simulink model "HANcoder_E407_CAN_COMM_TEST"  (R2018b)
settings: Solver=FixedStepDiscrete  StartTime=0.0  StopTime=1  FixedStep=0.01  RelTol=1e-3
PreLoadFcn:
  | librarySetup
  | eval([bdroot,'_startup']) %Calling [modelName]_startup.m
values from neighbouring files (symbols this model uses):
  HANtuneOverride = Simulink.Parameter    [HANcoder_E407_CAN_COMM_TEST_startup.m]    (also in HANcoder_E407_TTA_Controller_v3_startup.m; HANcoder_E407_TTA_Template_startup.m; HANcoder_Olimexino_startup.m)
  ID_CAN1_const = 24    [HANcoder_E407_CAN_COMM_TEST_startup.m]
  ID_CAN2_const = 24    [HANcoder_E407_CAN_COMM_TEST_startup.m]
  precision_CAN1 = Simulink.Parameter    [HANcoder_E407_CAN_COMM_TEST_startup.m]
  precision_CAN2 = Simulink.Parameter    [HANcoder_E407_CAN_COMM_TEST_startup.m]
  Rx_ID_CAN1 = Simulink.Parameter    [HANcoder_E407_CAN_COMM_TEST_startup.m]
  Rx_ID_CAN2 = Simulink.Parameter    [HANcoder_E407_CAN_COMM_TEST_startup.m]
  Tx_Buffer_1_CAN1 = Simulink.Parameter    [HANcoder_E407_CAN_COMM_TEST_startup.m]
  Tx_Buffer_1_CAN2 = Simulink.Parameter    [HANcoder_E407_CAN_COMM_TEST_startup.m]
  Tx_Buffer_2_CAN1 = Simulink.Parameter    [HANcoder_E407_CAN_COMM_TEST_startup.m]
  Tx_Buffer_2_CAN2 = Simulink.Parameter    [HANcoder_E407_CAN_COMM_TEST_startup.m]
  Tx_Buffer_3_CAN1 = Simulink.Parameter    [HANcoder_E407_CAN_COMM_TEST_startup.m]
  Tx_Buffer_3_CAN2 = Simulink.Parameter    [HANcoder_E407_CAN_COMM_TEST_startup.m]
  Tx_Buffer_4_CAN1 = Simulink.Parameter    [HANcoder_E407_CAN_COMM_TEST_startup.m]
  Tx_Buffer_4_CAN2 = Simulink.Parameter    [HANcoder_E407_CAN_COMM_TEST_startup.m]
  Tx_Buffer_5_CAN1 = Simulink.Parameter    [HANcoder_E407_CAN_COMM_TEST_startup.m]
  Tx_Buffer_5_CAN2 = Simulink.Parameter    [HANcoder_E407_CAN_COMM_TEST_startup.m]
  Tx_Buffer_6_CAN1 = Simulink.Parameter    [HANcoder_E407_CAN_COMM_TEST_startup.m]
  Tx_Buffer_6_CAN2 = Simulink.Parameter    [HANcoder_E407_CAN_COMM_TEST_startup.m]
  Tx_Buffer_7_CAN1 = Simulink.Parameter    [HANcoder_E407_CAN_COMM_TEST_startup.m]
  Tx_Buffer_7_CAN2 = Simulink.Parameter    [HANcoder_E407_CAN_COMM_TEST_startup.m]
  Tx_Buffer_8_CAN1 = Simulink.Parameter    [HANcoder_E407_CAN_COMM_TEST_startup.m]
  Tx_Buffer_8_CAN2 = Simulink.Parameter    [HANcoder_E407_CAN_COMM_TEST_startup.m]
  Tx_ID_CAN1 = Simulink.Parameter    [HANcoder_E407_CAN_COMM_TEST_startup.m]
  Tx_ID_CAN2 = Simulink.Parameter    [HANcoder_E407_CAN_COMM_TEST_startup.m]
  Tx_Max_CAN1 = Simulink.Parameter    [HANcoder_E407_CAN_COMM_TEST_startup.m]
  Tx_Max_CAN2 = Simulink.Parameter    [HANcoder_E407_CAN_COMM_TEST_startup.m]
  Tx_Min_CAN1 = Simulink.Parameter    [HANcoder_E407_CAN_COMM_TEST_startup.m]
  Tx_Min_CAN2 = Simulink.Parameter    [HANcoder_E407_CAN_COMM_TEST_startup.m]
libraries: hdlsllib x48, HANcoder_STM32_Target x13, simulink x2
(part 2 of 3)

== system HANcoder_E407_CAN_COMM_TEST/HANcoder STM32 Target - E407-STM32 algorithm/Rx CAN/uint8_2float4 ==
  precision : Inport
  value : Inport  Port=2
  Bit Shift : hdlsllib/Logic and Bit Operations/Bit Shift  mode=Shift Right Logical  N=7
      settings: SourceProductName=HDL Coder  SourceProductBaseCode=HD
  Bit Shift1 : hdlsllib/Logic and Bit Operations/Bit Shift  mode=Shift Left Logical  N=7
      settings: SourceProductName=HDL Coder  SourceProductBaseCode=HD
  Cast1 : DataTypeConversion  OutDataTypeStr=double
  Constant1 : Constant  Value=2
  Constant2 : Constant  Value=2
  Display{1..5} (5 alike) : Display
  Divide : Product  Inputs=*/
  Fix1 : Rounding  Operator=fix
  Gain : Gain  Gain=-1
  Gain1 : Gain  Gain=-1
  Minus : Sum  Inputs=-+
  Minus1 : Sum  Inputs=+-
  Minus2 : Sum
  Multiply : Product
  Multiply1 : Product
  Power : Math  Priority=5  Operator=pow  SaturateOnIntegerOverflow=on
  Power1 : Math  Priority=5  Operator=pow  SaturateOnIntegerOverflow=on
  Switch : Switch  Criteria=u2 > Threshold
  decoded : Outport
  wires:
  Bit Shift1/1 -> Minus/1
  [prec_pow] -> Multiply1/2
  [prec_pow] -> Divide/2
  Power1/1 -> [prec_pow]
  Constant2/1 -> Power1/1
  precision/1 -> [precision], Power1/2
  Cast1/1 -> Minus/2
  Divide/1 -> Fix1/1
  Switch/1 -> decoded/1, Display3/1
  Gain1/1 -> Switch/1
  Minus2/1 -> Switch/3, Gain1/1
  Multiply/1 -> Minus2/1
  [precision] -> Gain/1
  Power/1 -> Multiply/2
  Gain/1 -> Power/2
  Constant1/1 -> Power/1
  Minus1/1 -> Multiply/1, Display5/1
  Multiply1/1 -> Minus1/2
  Fix1/1 -> Multiply1/1, Display4/1, Minus2/2
  Minus/1 -> Minus1/1, Display2/1, Divide/1
  value/1 -> Bit Shift/1, Cast1/1
  Bit Shift/1 -> Display1/1, Switch/2, Bit Shift1/1

== system HANcoder_E407_CAN_COMM_TEST/HANcoder STM32 Target - E407-STM32 algorithm/Rx CAN/uint8_2float5 ==
  precision : Inport
  value : Inport  Port=2
  Bit Shift : hdlsllib/Logic and Bit Operations/Bit Shift  mode=Shift Right Logical  N=7
      settings: SourceProductName=HDL Coder  SourceProductBaseCode=HD
  Bit Shift1 : hdlsllib/Logic and Bit Operations/Bit Shift  mode=Shift Left Logical  N=7
      settings: SourceProductName=HDL Coder  SourceProductBaseCode=HD
  Cast1 : DataTypeConversion  OutDataTypeStr=double
  Constant1 : Constant  Value=2
  Constant2 : Constant  Value=2
  Display{1..5} (5 alike) : Display
  Divide : Product  Inputs=*/
  Fix1 : Rounding  Operator=fix
  Gain : Gain  Gain=-1
  Gain1 : Gain  Gain=-1
  Minus : Sum  Inputs=-+
  Minus1 : Sum  Inputs=+-
  Minus2 : Sum
  Multiply : Product
  Multiply1 : Product
  Power : Math  Priority=5  Operator=pow  SaturateOnIntegerOverflow=on
  Power1 : Math  Priority=5  Operator=pow  SaturateOnIntegerOverflow=on
  Switch : Switch  Criteria=u2 > Threshold
  decoded : Outport
  wires:
  Bit Shift/1 -> Bit Shift1/1, Switch/2, Display1/1
  value/1 -> Cast1/1, Bit Shift/1
  Minus/1 -> Divide/1, Display2/1, Minus1/1
  Fix1/1 -> Minus2/2, Display4/1, Multiply1/1
  Multiply1/1 -> Minus1/2
  Minus1/1 -> Display5/1, Multiply/1
  Constant1/1 -> Power/1
  Gain/1 -> Power/2
  Power/1 -> Multiply/2
  [precision] -> Gain/1
  Multiply/1 -> Minus2/1
  Minus2/1 -> Gain1/1, Switch/3
  Gain1/1 -> Switch/1
  Switch/1 -> Display3/1, decoded/1
  Divide/1 -> Fix1/1
  Cast1/1 -> Minus/2
  precision/1 -> Power1/2, [precision]
  Constant2/1 -> Power1/1
  Power1/1 -> [prec_pow]
  [prec_pow] -> Divide/2
  [prec_pow] -> Multiply1/2
  Bit Shift1/1 -> Minus/1

== system HANcoder_E407_CAN_COMM_TEST/HANcoder STM32 Target - E407-STM32 algorithm/Rx CAN/uint8_2float6 ==
  precision : Inport
  value : Inport  Port=2
  Bit Shift : hdlsllib/Logic and Bit Operations/Bit Shift  mode=Shift Right Logical  N=7
      settings: SourceProductName=HDL Coder  SourceProductBaseCode=HD
  Bit Shift1 : hdlsllib/Logic and Bit Operations/Bit Shift  mode=Shift Left Logical  N=7
      settings: SourceProductName=HDL Coder  SourceProductBaseCode=HD
  Cast1 : DataTypeConversion  OutDataTypeStr=double
  Constant1 : Constant  Value=2
  Constant2 : Constant  Value=2
  Display{1..5} (5 alike) : Display
  Divide : Product  Inputs=*/
  Fix1 : Rounding  Operator=fix
  Gain : Gain  Gain=-1
  Gain1 : Gain  Gain=-1
  Minus : Sum  Inputs=-+
  Minus1 : Sum  Inputs=+-
  Minus2 : Sum
  Multiply : Product
  Multiply1 : Product
  Power : Math  Priority=5  Operator=pow  SaturateOnIntegerOverflow=on
  Power1 : Math  Priority=5  Operator=pow  SaturateOnIntegerOverflow=on
  Switch : Switch  Criteria=u2 > Threshold
  decoded : Outport
  wires:
  Bit Shift1/1 -> Minus/1
  [prec_pow] -> Multiply1/2
  [prec_pow] -> Divide/2
  Power1/1 -> [prec_pow]
  Constant2/1 -> Power1/1
  precision/1 -> [precision], Power1/2
  Cast1/1 -> Minus/2
  Divide/1 -> Fix1/1
  Switch/1 -> decoded/1, Display3/1
  Gain1/1 -> Switch/1
  Minus2/1 -> Switch/3, Gain1/1
  Multiply/1 -> Minus2/1
  [precision] -> Gain/1
  Power/1 -> Multiply/2
  Gain/1 -> Power/2
  Constant1/1 -> Power/1
  Minus1/1 -> Multiply/1, Display5/1
  Multiply1/1 -> Minus1/2
  Fix1/1 -> Multiply1/1, Display4/1, Minus2/2
  Minus/1 -> Minus1/1, Display2/1, Divide/1
  value/1 -> Bit Shift/1, Cast1/1
  Bit Shift/1 -> Display1/1, Switch/2, Bit Shift1/1

== system HANcoder_E407_CAN_COMM_TEST/HANcoder STM32 Target - E407-STM32 algorithm/Rx CAN/uint8_2float7 ==
  precision : Inport
  value : Inport  Port=2
  Bit Shift : hdlsllib/Logic and Bit Operations/Bit Shift  mode=Shift Right Logical  N=7
      settings: SourceProductName=HDL Coder  SourceProductBaseCode=HD
  Bit Shift1 : hdlsllib/Logic and Bit Operations/Bit Shift  mode=Shift Left Logical  N=7
      settings: SourceProductName=HDL Coder  SourceProductBaseCode=HD
  Cast1 : DataTypeConversion  OutDataTypeStr=double
  Constant1 : Constant  Value=2
  Constant2 : Constant  Value=2
  Display{1..5} (5 alike) : Display
  Divide : Product  Inputs=*/
  Fix1 : Rounding  Operator=fix
  Gain : Gain  Gain=-1
  Gain1 : Gain  Gain=-1
  Minus : Sum  Inputs=-+
  Minus1 : Sum  Inputs=+-
  Minus2 : Sum
  Multiply : Product
  Multiply1 : Product
  Power : Math  Priority=5  Operator=pow  SaturateOnIntegerOverflow=on
  Power1 : Math  Priority=5  Operator=pow  SaturateOnIntegerOverflow=on
  Switch : Switch  Criteria=u2 > Threshold
  decoded : Outport
  wires:
  Bit Shift/1 -> Bit Shift1/1, Switch/2, Display1/1
  value/1 -> Cast1/1, Bit Shift/1
  Minus/1 -> Divide/1, Display2/1, Minus1/1
  Fix1/1 -> Minus2/2, Display4/1, Multiply1/1
  Multiply1/1 -> Minus1/2
  Minus1/1 -> Display5/1, Multiply/1
  Constant1/1 -> Power/1
  Gain/1 -> Power/2
  Power/1 -> Multiply/2
  [precision] -> Gain/1
  Multiply/1 -> Minus2/1
  Minus2/1 -> Gain1/1, Switch/3
  Gain1/1 -> Switch/1
  Switch/1 -> Display3/1, decoded/1
  Divide/1 -> Fix1/1
  Cast1/1 -> Minus/2
  precision/1 -> Power1/2, [precision]
  Constant2/1 -> Power1/1
  Power1/1 -> [prec_pow]
  [prec_pow] -> Divide/2
  [prec_pow] -> Multiply1/2
  Bit Shift1/1 -> Minus/1

== system HANcoder_E407_CAN_COMM_TEST/HANcoder STM32 Target - E407-STM32 algorithm/Rx CAN/uint8_2float8 ==
  precision : Inport
  value : Inport  Port=2
  Bit Shift : hdlsllib/Logic and Bit Operations/Bit Shift  mode=Shift Right Logical  N=7
      settings: SourceProductName=HDL Coder  SourceProductBaseCode=HD
  Bit Shift1 : hdlsllib/Logic and Bit Operations/Bit Shift  mode=Shift Left Logical  N=7
      settings: SourceProductName=HDL Coder  SourceProductBaseCode=HD
  Cast1 : DataTypeConversion  OutDataTypeStr=double
  Constant1 : Constant  Value=2
  Constant2 : Constant  Value=2
  Display{1..5} (5 alike) : Display
  Divide : Product  Inputs=*/
  Fix1 : Rounding  Operator=fix
  Gain : Gain  Gain=-1
  Gain1 : Gain  Gain=-1
  Minus : Sum  Inputs=-+
  Minus1 : Sum  Inputs=+-
  Minus2 : Sum
  Multiply : Product
  Multiply1 : Product
  Power : Math  Priority=5  Operator=pow  SaturateOnIntegerOverflow=on
  Power1 : Math  Priority=5  Operator=pow  SaturateOnIntegerOverflow=on
  Switch : Switch  Criteria=u2 > Threshold
  decoded : Outport
  wires:
  Bit Shift/1 -> Bit Shift1/1, Switch/2, Display1/1
  value/1 -> Cast1/1, Bit Shift/1
  Minus/1 -> Divide/1, Display2/1, Minus1/1
  Fix1/1 -> Minus2/2, Display4/1, Multiply1/1
  Multiply1/1 -> Minus1/2
  Minus1/1 -> Display5/1, Multiply/1
  Constant1/1 -> Power/1
  Gain/1 -> Power/2
  Power/1 -> Multiply/2
  [precision] -> Gain/1
  Multiply/1 -> Minus2/1
  Minus2/1 -> Gain1/1, Switch/3
  Gain1/1 -> Switch/1
  Switch/1 -> Display3/1, decoded/1
  Divide/1 -> Fix1/1
  Cast1/1 -> Minus/2
  precision/1 -> Power1/2, [precision]
  Constant2/1 -> Power1/1
  Power1/1 -> [prec_pow]
  [prec_pow] -> Divide/2
  [prec_pow] -> Multiply1/2
  Bit Shift1/1 -> Minus/1

== system HANcoder_E407_CAN_COMM_TEST/HANcoder STM32 Target - E407-STM32 algorithm/Rx CAN/uint8_2float9 ==
  precision : Inport
  value : Inport  Port=2
  Bit Shift : hdlsllib/Logic and Bit Operations/Bit Shift  mode=Shift Right Logical  N=7
      settings: SourceProductName=HDL Coder  SourceProductBaseCode=HD
  Bit Shift1 : hdlsllib/Logic and Bit Operations/Bit Shift  mode=Shift Left Logical  N=7
      settings: SourceProductName=HDL Coder  SourceProductBaseCode=HD
  Cast1 : DataTypeConversion  OutDataTypeStr=double
  Constant1 : Constant  Value=2
  Constant2 : Constant  Value=2
  Display{1..5} (5 alike) : Display
  Divide : Product  Inputs=*/
  Fix1 : Rounding  Operator=fix
  Gain : Gain  Gain=-1
  Gain1 : Gain  Gain=-1
  Minus : Sum  Inputs=-+
  Minus1 : Sum  Inputs=+-
  Minus2 : Sum
  Multiply : Product
  Multiply1 : Product
  Power : Math  Priority=5  Operator=pow  SaturateOnIntegerOverflow=on
  Power1 : Math  Priority=5  Operator=pow  SaturateOnIntegerOverflow=on
  Switch : Switch  Criteria=u2 > Threshold
  decoded : Outport
  wires:
  Bit Shift/1 -> Bit Shift1/1, Switch/2, Display1/1
  value/1 -> Cast1/1, Bit Shift/1
  Minus/1 -> Divide/1, Display2/1, Minus1/1
  Fix1/1 -> Minus2/2, Display4/1, Multiply1/1
  Multiply1/1 -> Minus1/2
  Minus1/1 -> Display5/1, Multiply/1
  Constant1/1 -> Power/1
  Gain/1 -> Power/2
  Power/1 -> Multiply/2
  [precision] -> Gain/1
  Multiply/1 -> Minus2/1
  Minus2/1 -> Gain1/1, Switch/3
  Gain1/1 -> Switch/1
  Switch/1 -> Display3/1, decoded/1
  Divide/1 -> Fix1/1
  Cast1/1 -> Minus/2
  precision/1 -> Power1/2, [precision]
  Constant2/1 -> Power1/1
  Power1/1 -> [prec_pow]
  [prec_pow] -> Divide/2
  [prec_pow] -> Multiply1/2
  Bit Shift1/1 -> Minus/1

== system HANcoder_E407_CAN_COMM_TEST/HANcoder STM32 Target - E407-STM32 algorithm/Tx CAN/CAN send ==
  In1 : Inport
  In2 : Inport  Port=2
  In3 : Inport  Port=3
  In4 : Inport  Port=4
  In5 : Inport  Port=5
  In6 : Inport  Port=6
  In7 : Inport  Port=7
  In8 : Inport  Port=8
  In9 : Inport  Port=9
  S-Function : M-S-Function  FunctionName=sfcn_can_send  Parameters=tsamp, canBus, frameType, inputNumber, dataType, byteOrder
  wires:
  In1/1 -> S-Function/1
  In2/1 -> S-Function/2
  In3/1 -> S-Function/3
  In4/1 -> S-Function/4
  In5/1 -> S-Function/5
  In6/1 -> S-Function/6
  In7/1 -> S-Function/7
  In8/1 -> S-Function/8
  In9/1 -> S-Function/9

== system HANcoder_E407_CAN_COMM_TEST/HANcoder STM32 Target - E407-STM32 algorithm/Tx CAN/CAN send1 ==
  In1 : Inport
  In2 : Inport  Port=2
  In3 : Inport  Port=3
  In4 : Inport  Port=4
  In5 : Inport  Port=5
  In6 : Inport  Port=6
  In7 : Inport  Port=7
  In8 : Inport  Port=8
  In9 : Inport  Port=9
  S-Function : M-S-Function  FunctionName=sfcn_can_send  Parameters=tsamp, canBus, frameType, inputNumber, dataType, byteOrder
  wires:
  In9/1 -> S-Function/9
  In8/1 -> S-Function/8
  In7/1 -> S-Function/7
  In6/1 -> S-Function/6
  In5/1 -> S-Function/5
  In4/1 -> S-Function/4
  In3/1 -> S-Function/3
  In2/1 -> S-Function/2
  In1/1 -> S-Function/1

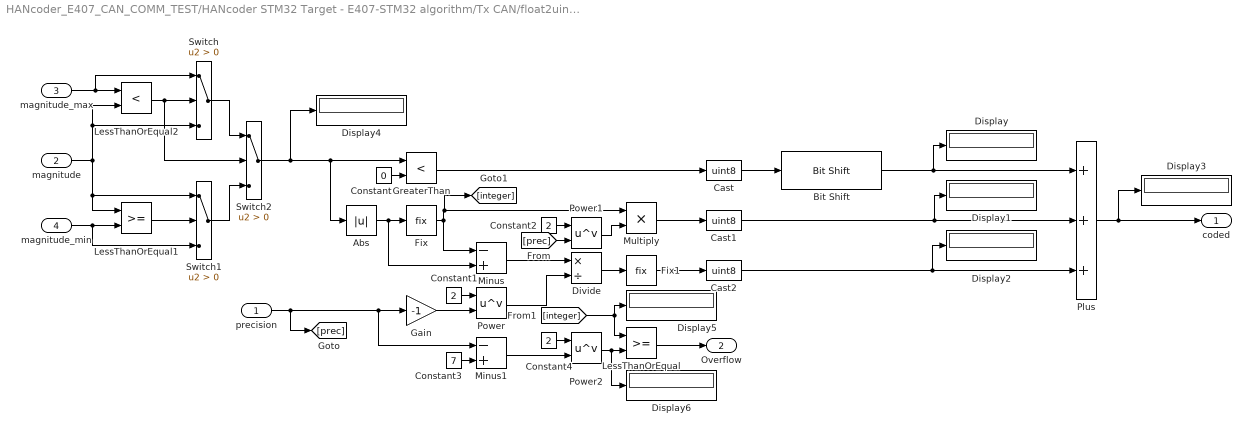
== system HANcoder_E407_CAN_COMM_TEST/HANcoder STM32 Target - E407-STM32 algorithm/Tx CAN/float2uint1 ==
  precision : Inport
  magnitude : Inport  Port=2
  magnitude_max : Inport  Port=3
  magnitude_min : Inport  Port=4
  Abs : Abs
  Bit Shift : hdlsllib/Logic and Bit Operations/Bit Shift  mode=Shift Left Logical  N=7
      settings: SourceProductName=HDL Coder  SourceProductBaseCode=HD
  Cast : DataTypeConversion  OutDataTypeStr=uint8
  Cast1 : DataTypeConversion  OutDataTypeStr=uint8
  Cast2 : DataTypeConversion  OutDataTypeStr=uint8
  Constant : Constant  Value=0
  Constant1 : Constant  Value=2
  Constant2 : Constant  Value=2
  Constant3 : Constant  Value=7
  Constant4 : Constant  Value=2
  Display{,1..6} (7 alike) : Display
  Divide : Product  Inputs=*/
  Fix : Rounding  Priority=3  Operator=fix
  Fix1 : Rounding  Priority=6  Operator=fix
  Gain : Gain  Gain=-1
  GreaterThan : RelationalOperator  Priority=2  Operator=<  OutDataTypeStr=boolean  RndMeth=Simplest
  LessThanOrEqual : RelationalOperator  OutDataTypeStr=boolean  RndMeth=Simplest
  LessThanOrEqual1 : RelationalOperator  OutDataTypeStr=boolean  RndMeth=Simplest
  LessThanOrEqual2 : RelationalOperator  Operator=<  OutDataTypeStr=boolean  RndMeth=Simplest
  Minus : Sum  Priority=4  Inputs=-+
  Minus1 : Sum  Priority=4  Inputs=-+
  Multiply : Product
  Plus : Sum  Priority=10  Inputs=+++
  Power : Math  Priority=5  Operator=pow  SaturateOnIntegerOverflow=on
  Power1 : Math  Priority=5  Operator=pow  SaturateOnIntegerOverflow=on
  Power2 : Math  Priority=5  Operator=pow  SaturateOnIntegerOverflow=on
  Switch : Switch  Criteria=u2 > Threshold
  Switch1 : Switch  Criteria=u2 > Threshold
  Switch2 : Switch  Criteria=u2 > Threshold
  coded : Outport
  Overflow : Outport  Port=2
  wires:
  Constant/1 -> GreaterThan/2
  Switch2/1 -> Display4/1, Abs/1, GreaterThan/1
  Abs/1 -> Minus/2, Fix/1
  GreaterThan/1 -> Cast/1
  Fix/1 -> [integer], Multiply/1, Minus/1
  Minus/1 -> Divide/1
  Cast/1 -> Bit Shift/1
  Bit Shift/1 -> Display/1, Plus/1
  Cast1/1 -> Display1/1, Plus/2
  Constant1/1 -> Power/1
  Gain/1 -> Power/2
  Power/1 -> Divide/2
  Divide/1 -> Fix1/1
  Fix1/1 -> Cast2/1
  Cast2/1 -> Display2/1, Plus/3
  Constant2/1 -> Power1/1
  Power1/1 -> Multiply/2
  precision/1 -> [prec], Minus1/1, Gain/1
  Multiply/1 -> Cast1/1
  [prec] -> Power1/2
  Constant3/1 -> Minus1/2
  Minus1/1 -> Power2/2
  Constant4/1 -> Power2/1
  Power2/1 -> Display6/1, LessThanOrEqual/2
  LessThanOrEqual/1 -> Overflow/1
  Plus/1 -> coded/1, Display3/1
  magnitude/1 -> LessThanOrEqual1/1, Switch1/1, LessThanOrEqual2/2, Switch/3
  magnitude_min/1 -> LessThanOrEqual1/2, Switch1/3
  magnitude_max/1 -> Switch/1, LessThanOrEqual2/1
  LessThanOrEqual2/1 -> Switch2/2, Switch/2
  LessThanOrEqual1/1 -> Switch1/2
  Switch/1 -> Switch2/1
  Switch1/1 -> Switch2/3
  [integer] -> Display5/1, LessThanOrEqual/1

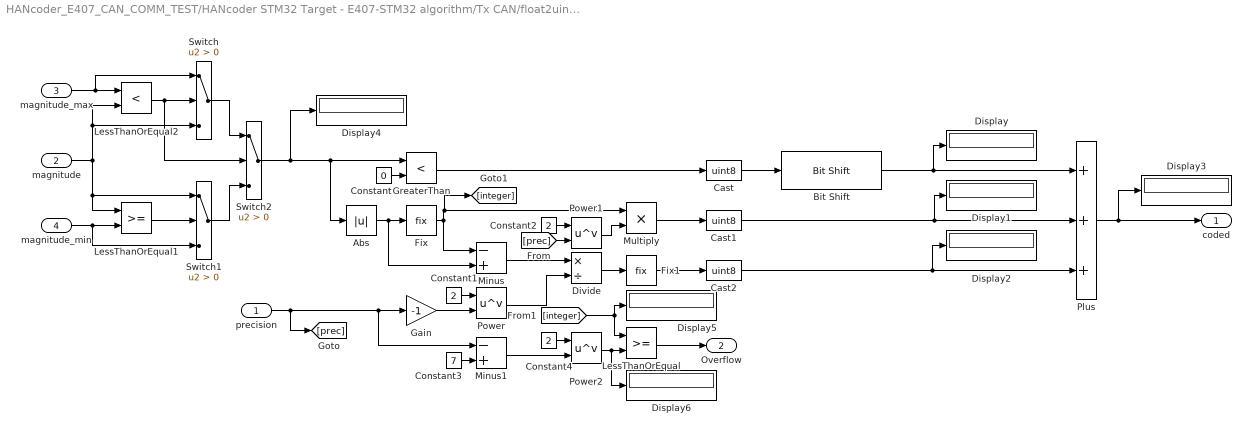
== system HANcoder_E407_CAN_COMM_TEST/HANcoder STM32 Target - E407-STM32 algorithm/Tx CAN/float2uint10 ==
  precision : Inport
  magnitude : Inport  Port=2
  magnitude_max : Inport  Port=3
  magnitude_min : Inport  Port=4
  Abs : Abs
  Bit Shift : hdlsllib/Logic and Bit Operations/Bit Shift  mode=Shift Left Logical  N=7
      settings: SourceProductName=HDL Coder  SourceProductBaseCode=HD
  Cast : DataTypeConversion  OutDataTypeStr=uint8
  Cast1 : DataTypeConversion  OutDataTypeStr=uint8
  Cast2 : DataTypeConversion  OutDataTypeStr=uint8
  Constant : Constant  Value=0
  Constant1 : Constant  Value=2
  Constant2 : Constant  Value=2
  Constant3 : Constant  Value=7
  Constant4 : Constant  Value=2
  Display{,1..6} (7 alike) : Display
  Divide : Product  Inputs=*/
  Fix : Rounding  Priority=3  Operator=fix
  Fix1 : Rounding  Priority=6  Operator=fix
  Gain : Gain  Gain=-1
  GreaterThan : RelationalOperator  Priority=2  Operator=<  OutDataTypeStr=boolean  RndMeth=Simplest
  LessThanOrEqual : RelationalOperator  OutDataTypeStr=boolean  RndMeth=Simplest
  LessThanOrEqual1 : RelationalOperator  OutDataTypeStr=boolean  RndMeth=Simplest
  LessThanOrEqual2 : RelationalOperator  Operator=<  OutDataTypeStr=boolean  RndMeth=Simplest
  Minus : Sum  Priority=4  Inputs=-+
  Minus1 : Sum  Priority=4  Inputs=-+
  Multiply : Product
  Plus : Sum  Priority=10  Inputs=+++
  Power : Math  Priority=5  Operator=pow  SaturateOnIntegerOverflow=on
  Power1 : Math  Priority=5  Operator=pow  SaturateOnIntegerOverflow=on
  Power2 : Math  Priority=5  Operator=pow  SaturateOnIntegerOverflow=on
  Switch : Switch  Criteria=u2 > Threshold
  Switch1 : Switch  Criteria=u2 > Threshold
  Switch2 : Switch  Criteria=u2 > Threshold
  coded : Outport
  Overflow : Outport  Port=2
  wires:
  Constant/1 -> GreaterThan/2
  Switch2/1 -> Display4/1, Abs/1, GreaterThan/1
  Abs/1 -> Minus/2, Fix/1
  GreaterThan/1 -> Cast/1
  Fix/1 -> [integer], Multiply/1, Minus/1
  Minus/1 -> Divide/1
  Cast/1 -> Bit Shift/1
  Bit Shift/1 -> Display/1, Plus/1
  Cast1/1 -> Display1/1, Plus/2
  Constant1/1 -> Power/1
  Gain/1 -> Power/2
  Power/1 -> Divide/2
  Divide/1 -> Fix1/1
  Fix1/1 -> Cast2/1
  Cast2/1 -> Display2/1, Plus/3
  Constant2/1 -> Power1/1
  Power1/1 -> Multiply/2
  precision/1 -> [prec], Minus1/1, Gain/1
  Multiply/1 -> Cast1/1
  [prec] -> Power1/2
  Constant3/1 -> Minus1/2
  Minus1/1 -> Power2/2
  Constant4/1 -> Power2/1
  Power2/1 -> Display6/1, LessThanOrEqual/2
  LessThanOrEqual/1 -> Overflow/1
  Plus/1 -> coded/1, Display3/1
  magnitude/1 -> LessThanOrEqual1/1, Switch1/1, LessThanOrEqual2/2, Switch/3
  magnitude_min/1 -> LessThanOrEqual1/2, Switch1/3
  magnitude_max/1 -> Switch/1, LessThanOrEqual2/1
  LessThanOrEqual2/1 -> Switch2/2, Switch/2
  LessThanOrEqual1/1 -> Switch1/2
  Switch/1 -> Switch2/1
  Switch1/1 -> Switch2/3
  [integer] -> Display5/1, LessThanOrEqual/1

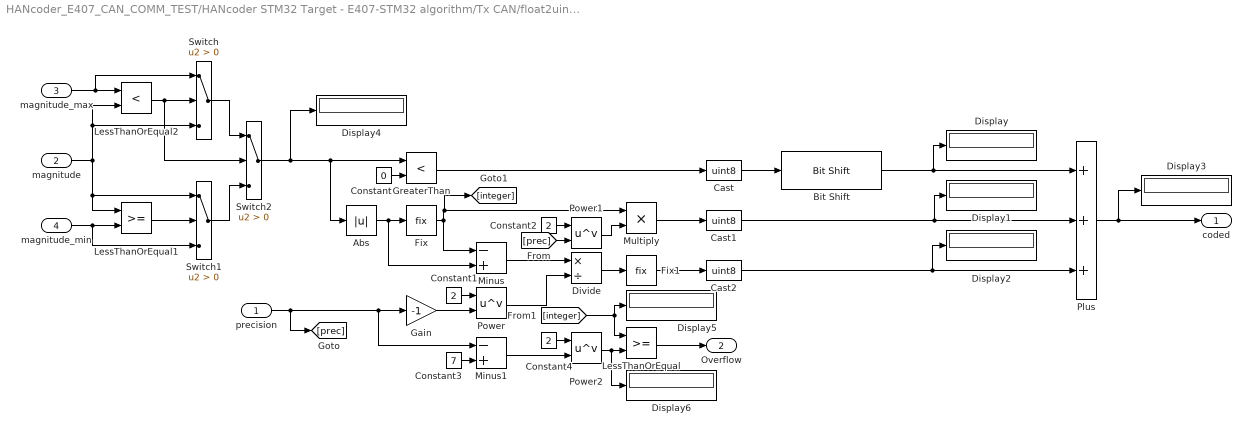
== system HANcoder_E407_CAN_COMM_TEST/HANcoder STM32 Target - E407-STM32 algorithm/Tx CAN/float2uint11 ==
  precision : Inport
  magnitude : Inport  Port=2
  magnitude_max : Inport  Port=3
  magnitude_min : Inport  Port=4
  Abs : Abs
  Bit Shift : hdlsllib/Logic and Bit Operations/Bit Shift  mode=Shift Left Logical  N=7
      settings: SourceProductName=HDL Coder  SourceProductBaseCode=HD
  Cast : DataTypeConversion  OutDataTypeStr=uint8
  Cast1 : DataTypeConversion  OutDataTypeStr=uint8
  Cast2 : DataTypeConversion  OutDataTypeStr=uint8
  Constant : Constant  Value=0
  Constant1 : Constant  Value=2
  Constant2 : Constant  Value=2
  Constant3 : Constant  Value=7
  Constant4 : Constant  Value=2
  Display{,1..6} (7 alike) : Display
  Divide : Product  Inputs=*/
  Fix : Rounding  Priority=3  Operator=fix
  Fix1 : Rounding  Priority=6  Operator=fix
  Gain : Gain  Gain=-1
  GreaterThan : RelationalOperator  Priority=2  Operator=<  OutDataTypeStr=boolean  RndMeth=Simplest
  LessThanOrEqual : RelationalOperator  OutDataTypeStr=boolean  RndMeth=Simplest
  LessThanOrEqual1 : RelationalOperator  OutDataTypeStr=boolean  RndMeth=Simplest
  LessThanOrEqual2 : RelationalOperator  Operator=<  OutDataTypeStr=boolean  RndMeth=Simplest
  Minus : Sum  Priority=4  Inputs=-+
  Minus1 : Sum  Priority=4  Inputs=-+
  Multiply : Product
  Plus : Sum  Priority=10  Inputs=+++
  Power : Math  Priority=5  Operator=pow  SaturateOnIntegerOverflow=on
  Power1 : Math  Priority=5  Operator=pow  SaturateOnIntegerOverflow=on
  Power2 : Math  Priority=5  Operator=pow  SaturateOnIntegerOverflow=on
  Switch : Switch  Criteria=u2 > Threshold
  Switch1 : Switch  Criteria=u2 > Threshold
  Switch2 : Switch  Criteria=u2 > Threshold
  coded : Outport
  Overflow : Outport  Port=2
  wires:
  [integer] -> LessThanOrEqual/1, Display5/1
  Switch1/1 -> Switch2/3
  Switch/1 -> Switch2/1
  LessThanOrEqual1/1 -> Switch1/2
  LessThanOrEqual2/1 -> Switch/2, Switch2/2
  magnitude_max/1 -> LessThanOrEqual2/1, Switch/1
  magnitude_min/1 -> Switch1/3, LessThanOrEqual1/2
  magnitude/1 -> Switch/3, LessThanOrEqual2/2, Switch1/1, LessThanOrEqual1/1
  Plus/1 -> Display3/1, coded/1
  LessThanOrEqual/1 -> Overflow/1
  Power2/1 -> LessThanOrEqual/2, Display6/1
  Constant4/1 -> Power2/1
  Minus1/1 -> Power2/2
  Constant3/1 -> Minus1/2
  [prec] -> Power1/2
  Multiply/1 -> Cast1/1
  precision/1 -> Gain/1, Minus1/1, [prec]
  Power1/1 -> Multiply/2
  Constant2/1 -> Power1/1
  Cast2/1 -> Plus/3, Display2/1
  Fix1/1 -> Cast2/1
  Divide/1 -> Fix1/1
  Power/1 -> Divide/2
  Gain/1 -> Power/2
  Constant1/1 -> Power/1
  Cast1/1 -> Plus/2, Display1/1
  Bit Shift/1 -> Plus/1, Display/1
  Cast/1 -> Bit Shift/1
  Minus/1 -> Divide/1
  Fix/1 -> Minus/1, Multiply/1, [integer]
  GreaterThan/1 -> Cast/1
  Abs/1 -> Fix/1, Minus/2
  Switch2/1 -> GreaterThan/1, Abs/1, Display4/1
  Constant/1 -> GreaterThan/2

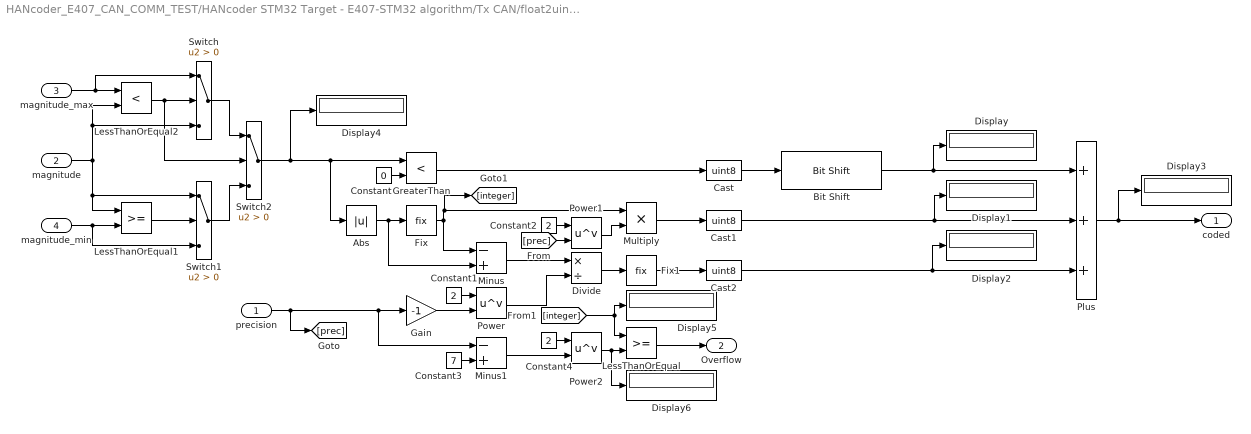
== system HANcoder_E407_CAN_COMM_TEST/HANcoder STM32 Target - E407-STM32 algorithm/Tx CAN/float2uint12 ==
  precision : Inport
  magnitude : Inport  Port=2
  magnitude_max : Inport  Port=3
  magnitude_min : Inport  Port=4
  Abs : Abs
  Bit Shift : hdlsllib/Logic and Bit Operations/Bit Shift  mode=Shift Left Logical  N=7
      settings: SourceProductName=HDL Coder  SourceProductBaseCode=HD
  Cast : DataTypeConversion  OutDataTypeStr=uint8
  Cast1 : DataTypeConversion  OutDataTypeStr=uint8
  Cast2 : DataTypeConversion  OutDataTypeStr=uint8
  Constant : Constant  Value=0
  Constant1 : Constant  Value=2
  Constant2 : Constant  Value=2
  Constant3 : Constant  Value=7
  Constant4 : Constant  Value=2
  Display{,1..6} (7 alike) : Display
  Divide : Product  Inputs=*/
  Fix : Rounding  Priority=3  Operator=fix
  Fix1 : Rounding  Priority=6  Operator=fix
  Gain : Gain  Gain=-1
  GreaterThan : RelationalOperator  Priority=2  Operator=<  OutDataTypeStr=boolean  RndMeth=Simplest
  LessThanOrEqual : RelationalOperator  OutDataTypeStr=boolean  RndMeth=Simplest
  LessThanOrEqual1 : RelationalOperator  OutDataTypeStr=boolean  RndMeth=Simplest
  LessThanOrEqual2 : RelationalOperator  Operator=<  OutDataTypeStr=boolean  RndMeth=Simplest
  Minus : Sum  Priority=4  Inputs=-+
  Minus1 : Sum  Priority=4  Inputs=-+
  Multiply : Product
  Plus : Sum  Priority=10  Inputs=+++
  Power : Math  Priority=5  Operator=pow  SaturateOnIntegerOverflow=on
  Power1 : Math  Priority=5  Operator=pow  SaturateOnIntegerOverflow=on
  Power2 : Math  Priority=5  Operator=pow  SaturateOnIntegerOverflow=on
  Switch : Switch  Criteria=u2 > Threshold
  Switch1 : Switch  Criteria=u2 > Threshold
  Switch2 : Switch  Criteria=u2 > Threshold
  coded : Outport
  Overflow : Outport  Port=2
  wires:
  Constant/1 -> GreaterThan/2
  Switch2/1 -> Display4/1, Abs/1, GreaterThan/1
  Abs/1 -> Minus/2, Fix/1
  GreaterThan/1 -> Cast/1
  Fix/1 -> [integer], Multiply/1, Minus/1
  Minus/1 -> Divide/1
  Cast/1 -> Bit Shift/1
  Bit Shift/1 -> Display/1, Plus/1
  Cast1/1 -> Display1/1, Plus/2
  Constant1/1 -> Power/1
  Gain/1 -> Power/2
  Power/1 -> Divide/2
  Divide/1 -> Fix1/1
  Fix1/1 -> Cast2/1
  Cast2/1 -> Display2/1, Plus/3
  Constant2/1 -> Power1/1
  Power1/1 -> Multiply/2
  precision/1 -> [prec], Minus1/1, Gain/1
  Multiply/1 -> Cast1/1
  [prec] -> Power1/2
  Constant3/1 -> Minus1/2
  Minus1/1 -> Power2/2
  Constant4/1 -> Power2/1
  Power2/1 -> Display6/1, LessThanOrEqual/2
  LessThanOrEqual/1 -> Overflow/1
  Plus/1 -> coded/1, Display3/1
  magnitude/1 -> LessThanOrEqual1/1, Switch1/1, LessThanOrEqual2/2, Switch/3
  magnitude_min/1 -> LessThanOrEqual1/2, Switch1/3
  magnitude_max/1 -> Switch/1, LessThanOrEqual2/1
  LessThanOrEqual2/1 -> Switch2/2, Switch/2
  LessThanOrEqual1/1 -> Switch1/2
  Switch/1 -> Switch2/1
  Switch1/1 -> Switch2/3
  [integer] -> Display5/1, LessThanOrEqual/1

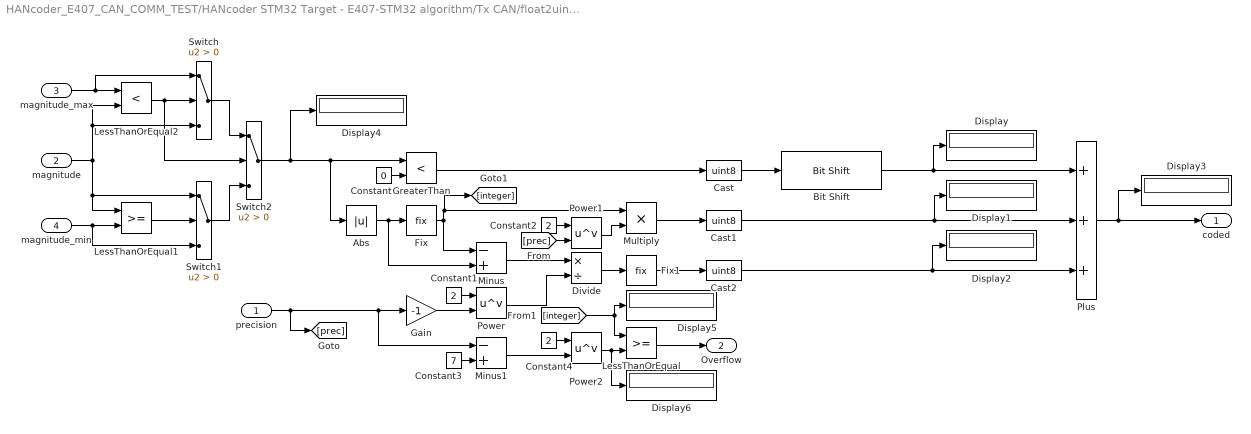
== system HANcoder_E407_CAN_COMM_TEST/HANcoder STM32 Target - E407-STM32 algorithm/Tx CAN/float2uint13 ==
  precision : Inport
  magnitude : Inport  Port=2
  magnitude_max : Inport  Port=3
  magnitude_min : Inport  Port=4
  Abs : Abs
  Bit Shift : hdlsllib/Logic and Bit Operations/Bit Shift  mode=Shift Left Logical  N=7
      settings: SourceProductName=HDL Coder  SourceProductBaseCode=HD
  Cast : DataTypeConversion  OutDataTypeStr=uint8
  Cast1 : DataTypeConversion  OutDataTypeStr=uint8
  Cast2 : DataTypeConversion  OutDataTypeStr=uint8
  Constant : Constant  Value=0
  Constant1 : Constant  Value=2
  Constant2 : Constant  Value=2
  Constant3 : Constant  Value=7
  Constant4 : Constant  Value=2
  Display{,1..6} (7 alike) : Display
  Divide : Product  Inputs=*/
  Fix : Rounding  Priority=3  Operator=fix
  Fix1 : Rounding  Priority=6  Operator=fix
  Gain : Gain  Gain=-1
  GreaterThan : RelationalOperator  Priority=2  Operator=<  OutDataTypeStr=boolean  RndMeth=Simplest
  LessThanOrEqual : RelationalOperator  OutDataTypeStr=boolean  RndMeth=Simplest
  LessThanOrEqual1 : RelationalOperator  OutDataTypeStr=boolean  RndMeth=Simplest
  LessThanOrEqual2 : RelationalOperator  Operator=<  OutDataTypeStr=boolean  RndMeth=Simplest
  Minus : Sum  Priority=4  Inputs=-+
  Minus1 : Sum  Priority=4  Inputs=-+
  Multiply : Product
  Plus : Sum  Priority=10  Inputs=+++
  Power : Math  Priority=5  Operator=pow  SaturateOnIntegerOverflow=on
  Power1 : Math  Priority=5  Operator=pow  SaturateOnIntegerOverflow=on
  Power2 : Math  Priority=5  Operator=pow  SaturateOnIntegerOverflow=on
  Switch : Switch  Criteria=u2 > Threshold
  Switch1 : Switch  Criteria=u2 > Threshold
  Switch2 : Switch  Criteria=u2 > Threshold
  coded : Outport
  Overflow : Outport  Port=2
  wires:
  [integer] -> LessThanOrEqual/1, Display5/1
  Switch1/1 -> Switch2/3
  Switch/1 -> Switch2/1
  LessThanOrEqual1/1 -> Switch1/2
  LessThanOrEqual2/1 -> Switch/2, Switch2/2
  magnitude_max/1 -> LessThanOrEqual2/1, Switch/1
  magnitude_min/1 -> Switch1/3, LessThanOrEqual1/2
  magnitude/1 -> Switch/3, LessThanOrEqual2/2, Switch1/1, LessThanOrEqual1/1
  Plus/1 -> Display3/1, coded/1
  LessThanOrEqual/1 -> Overflow/1
  Power2/1 -> LessThanOrEqual/2, Display6/1
  Constant4/1 -> Power2/1
  Minus1/1 -> Power2/2
  Constant3/1 -> Minus1/2
  [prec] -> Power1/2
  Multiply/1 -> Cast1/1
  precision/1 -> Gain/1, Minus1/1, [prec]
  Power1/1 -> Multiply/2
  Constant2/1 -> Power1/1
  Cast2/1 -> Plus/3, Display2/1
  Fix1/1 -> Cast2/1
  Divide/1 -> Fix1/1
  Power/1 -> Divide/2
  Gain/1 -> Power/2
  Constant1/1 -> Power/1
  Cast1/1 -> Plus/2, Display1/1
  Bit Shift/1 -> Plus/1, Display/1
  Cast/1 -> Bit Shift/1
  Minus/1 -> Divide/1
  Fix/1 -> Minus/1, Multiply/1, [integer]
  GreaterThan/1 -> Cast/1
  Abs/1 -> Fix/1, Minus/2
  Switch2/1 -> GreaterThan/1, Abs/1, Display4/1
  Constant/1 -> GreaterThan/2

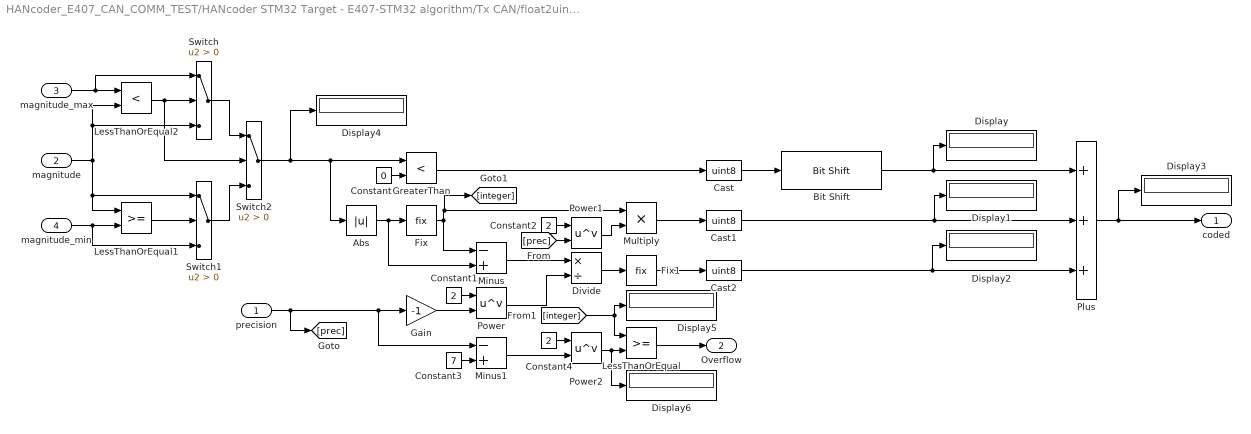
== system HANcoder_E407_CAN_COMM_TEST/HANcoder STM32 Target - E407-STM32 algorithm/Tx CAN/float2uint14 ==
  precision : Inport
  magnitude : Inport  Port=2
  magnitude_max : Inport  Port=3
  magnitude_min : Inport  Port=4
  Abs : Abs
  Bit Shift : hdlsllib/Logic and Bit Operations/Bit Shift  mode=Shift Left Logical  N=7
      settings: SourceProductName=HDL Coder  SourceProductBaseCode=HD
  Cast : DataTypeConversion  OutDataTypeStr=uint8
  Cast1 : DataTypeConversion  OutDataTypeStr=uint8
  Cast2 : DataTypeConversion  OutDataTypeStr=uint8
  Constant : Constant  Value=0
  Constant1 : Constant  Value=2
  Constant2 : Constant  Value=2
  Constant3 : Constant  Value=7
  Constant4 : Constant  Value=2
  Display{,1..6} (7 alike) : Display
  Divide : Product  Inputs=*/
  Fix : Rounding  Priority=3  Operator=fix
  Fix1 : Rounding  Priority=6  Operator=fix
  Gain : Gain  Gain=-1
  GreaterThan : RelationalOperator  Priority=2  Operator=<  OutDataTypeStr=boolean  RndMeth=Simplest
  LessThanOrEqual : RelationalOperator  OutDataTypeStr=boolean  RndMeth=Simplest
  LessThanOrEqual1 : RelationalOperator  OutDataTypeStr=boolean  RndMeth=Simplest
  LessThanOrEqual2 : RelationalOperator  Operator=<  OutDataTypeStr=boolean  RndMeth=Simplest
  Minus : Sum  Priority=4  Inputs=-+
  Minus1 : Sum  Priority=4  Inputs=-+
  Multiply : Product
  Plus : Sum  Priority=10  Inputs=+++
  Power : Math  Priority=5  Operator=pow  SaturateOnIntegerOverflow=on
  Power1 : Math  Priority=5  Operator=pow  SaturateOnIntegerOverflow=on
  Power2 : Math  Priority=5  Operator=pow  SaturateOnIntegerOverflow=on
  Switch : Switch  Criteria=u2 > Threshold
  Switch1 : Switch  Criteria=u2 > Threshold
  Switch2 : Switch  Criteria=u2 > Threshold
  coded : Outport
  Overflow : Outport  Port=2
  wires:
  Constant/1 -> GreaterThan/2
  Switch2/1 -> Display4/1, Abs/1, GreaterThan/1
  Abs/1 -> Minus/2, Fix/1
  GreaterThan/1 -> Cast/1
  Fix/1 -> [integer], Multiply/1, Minus/1
  Minus/1 -> Divide/1
  Cast/1 -> Bit Shift/1
  Bit Shift/1 -> Display/1, Plus/1
  Cast1/1 -> Display1/1, Plus/2
  Constant1/1 -> Power/1
  Gain/1 -> Power/2
  Power/1 -> Divide/2
  Divide/1 -> Fix1/1
  Fix1/1 -> Cast2/1
  Cast2/1 -> Display2/1, Plus/3
  Constant2/1 -> Power1/1
  Power1/1 -> Multiply/2
  precision/1 -> [prec], Minus1/1, Gain/1
  Multiply/1 -> Cast1/1
  [prec] -> Power1/2
  Constant3/1 -> Minus1/2
  Minus1/1 -> Power2/2
  Constant4/1 -> Power2/1
  Power2/1 -> Display6/1, LessThanOrEqual/2
  LessThanOrEqual/1 -> Overflow/1
  Plus/1 -> coded/1, Display3/1
  magnitude/1 -> LessThanOrEqual1/1, Switch1/1, LessThanOrEqual2/2, Switch/3
  magnitude_min/1 -> LessThanOrEqual1/2, Switch1/3
  magnitude_max/1 -> Switch/1, LessThanOrEqual2/1
  LessThanOrEqual2/1 -> Switch2/2, Switch/2
  LessThanOrEqual1/1 -> Switch1/2
  Switch/1 -> Switch2/1
  Switch1/1 -> Switch2/3
  [integer] -> Display5/1, LessThanOrEqual/1

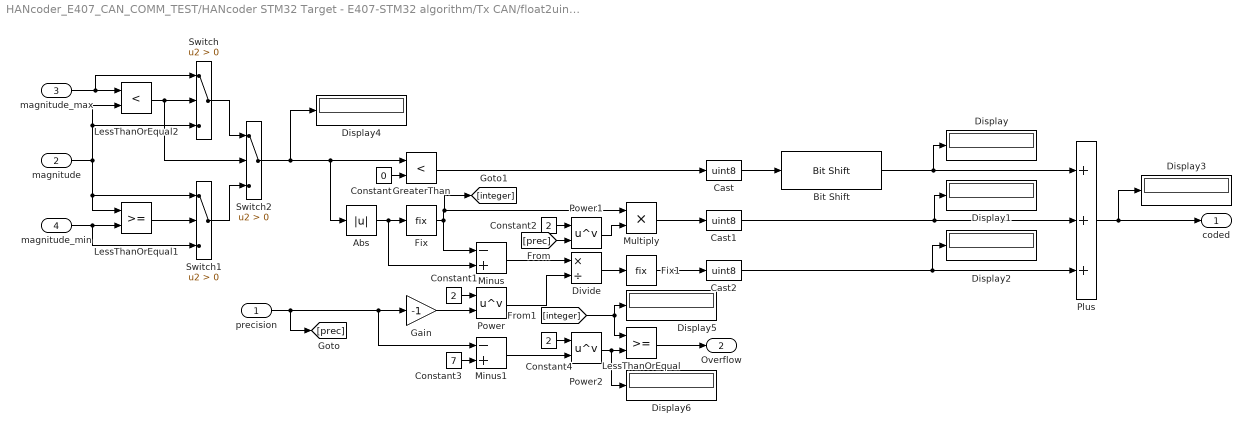
== system HANcoder_E407_CAN_COMM_TEST/HANcoder STM32 Target - E407-STM32 algorithm/Tx CAN/float2uint15 ==
  precision : Inport
  magnitude : Inport  Port=2
  magnitude_max : Inport  Port=3
  magnitude_min : Inport  Port=4
  Abs : Abs
  Bit Shift : hdlsllib/Logic and Bit Operations/Bit Shift  mode=Shift Left Logical  N=7
      settings: SourceProductName=HDL Coder  SourceProductBaseCode=HD
  Cast : DataTypeConversion  OutDataTypeStr=uint8
  Cast1 : DataTypeConversion  OutDataTypeStr=uint8
  Cast2 : DataTypeConversion  OutDataTypeStr=uint8
  Constant : Constant  Value=0
  Constant1 : Constant  Value=2
  Constant2 : Constant  Value=2
  Constant3 : Constant  Value=7
  Constant4 : Constant  Value=2
  Display{,1..6} (7 alike) : Display
  Divide : Product  Inputs=*/
  Fix : Rounding  Priority=3  Operator=fix
  Fix1 : Rounding  Priority=6  Operator=fix
  Gain : Gain  Gain=-1
  GreaterThan : RelationalOperator  Priority=2  Operator=<  OutDataTypeStr=boolean  RndMeth=Simplest
  LessThanOrEqual : RelationalOperator  OutDataTypeStr=boolean  RndMeth=Simplest
  LessThanOrEqual1 : RelationalOperator  OutDataTypeStr=boolean  RndMeth=Simplest
  LessThanOrEqual2 : RelationalOperator  Operator=<  OutDataTypeStr=boolean  RndMeth=Simplest
  Minus : Sum  Priority=4  Inputs=-+
  Minus1 : Sum  Priority=4  Inputs=-+
  Multiply : Product
  Plus : Sum  Priority=10  Inputs=+++
  Power : Math  Priority=5  Operator=pow  SaturateOnIntegerOverflow=on
  Power1 : Math  Priority=5  Operator=pow  SaturateOnIntegerOverflow=on
  Power2 : Math  Priority=5  Operator=pow  SaturateOnIntegerOverflow=on
  Switch : Switch  Criteria=u2 > Threshold
  Switch1 : Switch  Criteria=u2 > Threshold
  Switch2 : Switch  Criteria=u2 > Threshold
  coded : Outport
  Overflow : Outport  Port=2
  wires:
  [integer] -> LessThanOrEqual/1, Display5/1
  Switch1/1 -> Switch2/3
  Switch/1 -> Switch2/1
  LessThanOrEqual1/1 -> Switch1/2
  LessThanOrEqual2/1 -> Switch/2, Switch2/2
  magnitude_max/1 -> LessThanOrEqual2/1, Switch/1
  magnitude_min/1 -> Switch1/3, LessThanOrEqual1/2
  magnitude/1 -> Switch/3, LessThanOrEqual2/2, Switch1/1, LessThanOrEqual1/1
  Plus/1 -> Display3/1, coded/1
  LessThanOrEqual/1 -> Overflow/1
  Power2/1 -> LessThanOrEqual/2, Display6/1
  Constant4/1 -> Power2/1
  Minus1/1 -> Power2/2
  Constant3/1 -> Minus1/2
  [prec] -> Power1/2
  Multiply/1 -> Cast1/1
  precision/1 -> Gain/1, Minus1/1, [prec]
  Power1/1 -> Multiply/2
  Constant2/1 -> Power1/1
  Cast2/1 -> Plus/3, Display2/1
  Fix1/1 -> Cast2/1
  Divide/1 -> Fix1/1
  Power/1 -> Divide/2
  Gain/1 -> Power/2
  Constant1/1 -> Power/1
  Cast1/1 -> Plus/2, Display1/1
  Bit Shift/1 -> Plus/1, Display/1
  Cast/1 -> Bit Shift/1
  Minus/1 -> Divide/1
  Fix/1 -> Minus/1, Multiply/1, [integer]
  GreaterThan/1 -> Cast/1
  Abs/1 -> Fix/1, Minus/2
  Switch2/1 -> GreaterThan/1, Abs/1, Display4/1
  Constant/1 -> GreaterThan/2

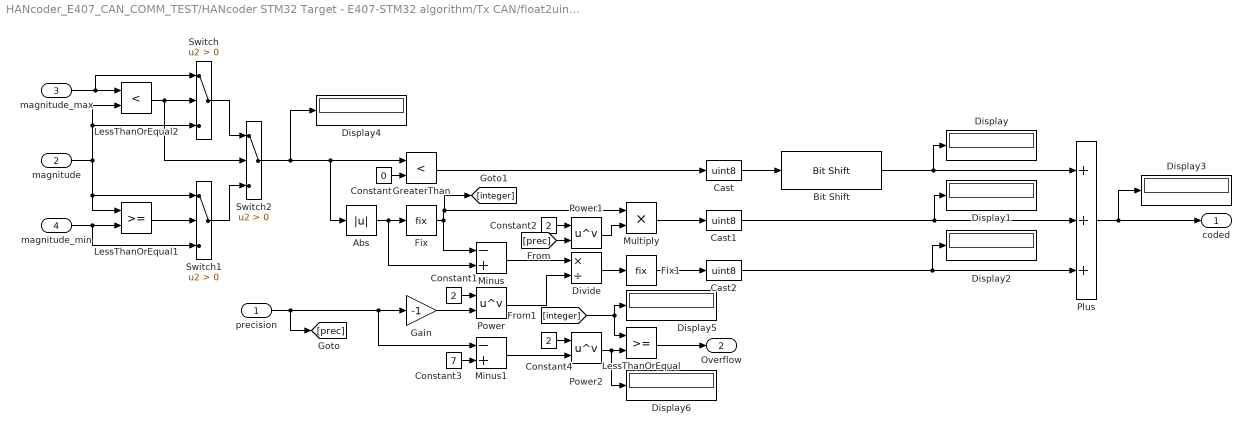
== system HANcoder_E407_CAN_COMM_TEST/HANcoder STM32 Target - E407-STM32 algorithm/Tx CAN/float2uint16 ==
  precision : Inport
  magnitude : Inport  Port=2
  magnitude_max : Inport  Port=3
  magnitude_min : Inport  Port=4
  Abs : Abs
  Bit Shift : hdlsllib/Logic and Bit Operations/Bit Shift  mode=Shift Left Logical  N=7
      settings: SourceProductName=HDL Coder  SourceProductBaseCode=HD
  Cast : DataTypeConversion  OutDataTypeStr=uint8
  Cast1 : DataTypeConversion  OutDataTypeStr=uint8
  Cast2 : DataTypeConversion  OutDataTypeStr=uint8
  Constant : Constant  Value=0
  Constant1 : Constant  Value=2
  Constant2 : Constant  Value=2
  Constant3 : Constant  Value=7
  Constant4 : Constant  Value=2
  Display{,1..6} (7 alike) : Display
  Divide : Product  Inputs=*/
  Fix : Rounding  Priority=3  Operator=fix
  Fix1 : Rounding  Priority=6  Operator=fix
  Gain : Gain  Gain=-1
  GreaterThan : RelationalOperator  Priority=2  Operator=<  OutDataTypeStr=boolean  RndMeth=Simplest
  LessThanOrEqual : RelationalOperator  OutDataTypeStr=boolean  RndMeth=Simplest
  LessThanOrEqual1 : RelationalOperator  OutDataTypeStr=boolean  RndMeth=Simplest
  LessThanOrEqual2 : RelationalOperator  Operator=<  OutDataTypeStr=boolean  RndMeth=Simplest
  Minus : Sum  Priority=4  Inputs=-+
  Minus1 : Sum  Priority=4  Inputs=-+
  Multiply : Product
  Plus : Sum  Priority=10  Inputs=+++
  Power : Math  Priority=5  Operator=pow  SaturateOnIntegerOverflow=on
  Power1 : Math  Priority=5  Operator=pow  SaturateOnIntegerOverflow=on
  Power2 : Math  Priority=5  Operator=pow  SaturateOnIntegerOverflow=on
  Switch : Switch  Criteria=u2 > Threshold
  Switch1 : Switch  Criteria=u2 > Threshold
  Switch2 : Switch  Criteria=u2 > Threshold
  coded : Outport
  Overflow : Outport  Port=2
  wires:
  Constant/1 -> GreaterThan/2
  Switch2/1 -> Display4/1, Abs/1, GreaterThan/1
  Abs/1 -> Minus/2, Fix/1
  GreaterThan/1 -> Cast/1
  Fix/1 -> [integer], Multiply/1, Minus/1
  Minus/1 -> Divide/1
  Cast/1 -> Bit Shift/1
  Bit Shift/1 -> Display/1, Plus/1
  Cast1/1 -> Display1/1, Plus/2
  Constant1/1 -> Power/1
  Gain/1 -> Power/2
  Power/1 -> Divide/2
  Divide/1 -> Fix1/1
  Fix1/1 -> Cast2/1
  Cast2/1 -> Display2/1, Plus/3
  Constant2/1 -> Power1/1
  Power1/1 -> Multiply/2
  precision/1 -> [prec], Minus1/1, Gain/1
  Multiply/1 -> Cast1/1
  [prec] -> Power1/2
  Constant3/1 -> Minus1/2
  Minus1/1 -> Power2/2
  Constant4/1 -> Power2/1
  Power2/1 -> Display6/1, LessThanOrEqual/2
  LessThanOrEqual/1 -> Overflow/1
  Plus/1 -> coded/1, Display3/1
  magnitude/1 -> LessThanOrEqual1/1, Switch1/1, LessThanOrEqual2/2, Switch/3
  magnitude_min/1 -> LessThanOrEqual1/2, Switch1/3
  magnitude_max/1 -> Switch/1, LessThanOrEqual2/1
  LessThanOrEqual2/1 -> Switch2/2, Switch/2
  LessThanOrEqual1/1 -> Switch1/2
  Switch/1 -> Switch2/1
  Switch1/1 -> Switch2/3
  [integer] -> Display5/1, LessThanOrEqual/1

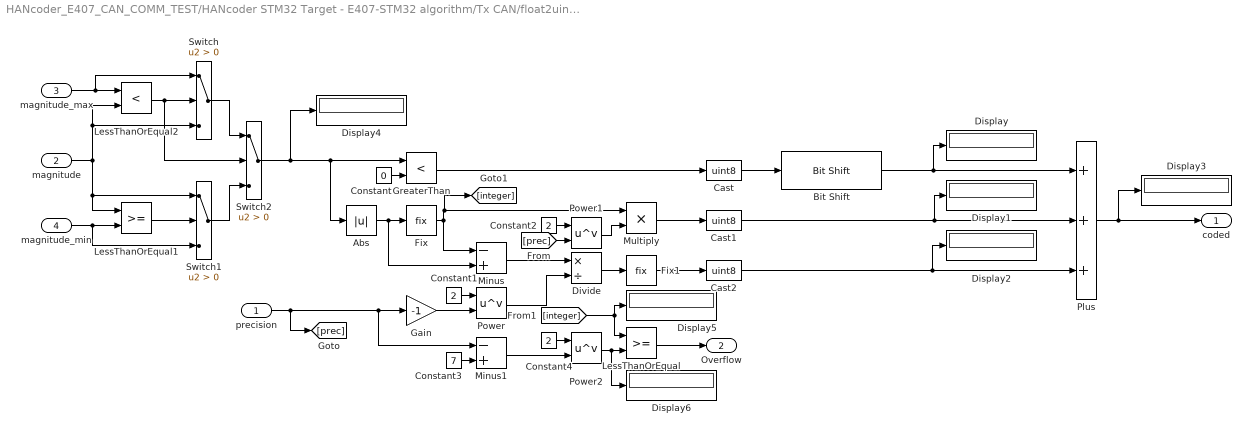
== system HANcoder_E407_CAN_COMM_TEST/HANcoder STM32 Target - E407-STM32 algorithm/Tx CAN/float2uint2 ==
  precision : Inport
  magnitude : Inport  Port=2
  magnitude_max : Inport  Port=3
  magnitude_min : Inport  Port=4
  Abs : Abs
  Bit Shift : hdlsllib/Logic and Bit Operations/Bit Shift  mode=Shift Left Logical  N=7
      settings: SourceProductName=HDL Coder  SourceProductBaseCode=HD
  Cast : DataTypeConversion  OutDataTypeStr=uint8
  Cast1 : DataTypeConversion  OutDataTypeStr=uint8
  Cast2 : DataTypeConversion  OutDataTypeStr=uint8
  Constant : Constant  Value=0
  Constant1 : Constant  Value=2
  Constant2 : Constant  Value=2
  Constant3 : Constant  Value=7
  Constant4 : Constant  Value=2
  Display{,1..6} (7 alike) : Display
  Divide : Product  Inputs=*/
  Fix : Rounding  Priority=3  Operator=fix
  Fix1 : Rounding  Priority=6  Operator=fix
  Gain : Gain  Gain=-1
  GreaterThan : RelationalOperator  Priority=2  Operator=<  OutDataTypeStr=boolean  RndMeth=Simplest
  LessThanOrEqual : RelationalOperator  OutDataTypeStr=boolean  RndMeth=Simplest
  LessThanOrEqual1 : RelationalOperator  OutDataTypeStr=boolean  RndMeth=Simplest
  LessThanOrEqual2 : RelationalOperator  Operator=<  OutDataTypeStr=boolean  RndMeth=Simplest
  Minus : Sum  Priority=4  Inputs=-+
  Minus1 : Sum  Priority=4  Inputs=-+
  Multiply : Product
  Plus : Sum  Priority=10  Inputs=+++
  Power : Math  Priority=5  Operator=pow  SaturateOnIntegerOverflow=on
  Power1 : Math  Priority=5  Operator=pow  SaturateOnIntegerOverflow=on
  Power2 : Math  Priority=5  Operator=pow  SaturateOnIntegerOverflow=on
  Switch : Switch  Criteria=u2 > Threshold
  Switch1 : Switch  Criteria=u2 > Threshold
  Switch2 : Switch  Criteria=u2 > Threshold
  coded : Outport
  Overflow : Outport  Port=2
  wires:
  [integer] -> LessThanOrEqual/1, Display5/1
  Switch1/1 -> Switch2/3
  Switch/1 -> Switch2/1
  LessThanOrEqual1/1 -> Switch1/2
  LessThanOrEqual2/1 -> Switch/2, Switch2/2
  magnitude_max/1 -> LessThanOrEqual2/1, Switch/1
  magnitude_min/1 -> Switch1/3, LessThanOrEqual1/2
  magnitude/1 -> Switch/3, LessThanOrEqual2/2, Switch1/1, LessThanOrEqual1/1
  Plus/1 -> Display3/1, coded/1
  LessThanOrEqual/1 -> Overflow/1
  Power2/1 -> LessThanOrEqual/2, Display6/1
  Constant4/1 -> Power2/1
  Minus1/1 -> Power2/2
  Constant3/1 -> Minus1/2
  [prec] -> Power1/2
  Multiply/1 -> Cast1/1
  precision/1 -> Gain/1, Minus1/1, [prec]
  Power1/1 -> Multiply/2
  Constant2/1 -> Power1/1
  Cast2/1 -> Plus/3, Display2/1
  Fix1/1 -> Cast2/1
  Divide/1 -> Fix1/1
  Power/1 -> Divide/2
  Gain/1 -> Power/2
  Constant1/1 -> Power/1
  Cast1/1 -> Plus/2, Display1/1
  Bit Shift/1 -> Plus/1, Display/1
  Cast/1 -> Bit Shift/1
  Minus/1 -> Divide/1
  Fix/1 -> Minus/1, Multiply/1, [integer]
  GreaterThan/1 -> Cast/1
  Abs/1 -> Fix/1, Minus/2
  Switch2/1 -> GreaterThan/1, Abs/1, Display4/1
  Constant/1 -> GreaterThan/2

== system HANcoder_E407_CAN_COMM_TEST/HANcoder STM32 Target - E407-STM32 algorithm/Tx CAN/float2uint3 ==
  precision : Inport
  magnitude : Inport  Port=2
  magnitude_max : Inport  Port=3
  magnitude_min : Inport  Port=4
  Abs : Abs
  Bit Shift : hdlsllib/Logic and Bit Operations/Bit Shift  mode=Shift Left Logical  N=7
      settings: SourceProductName=HDL Coder  SourceProductBaseCode=HD
  Cast : DataTypeConversion  OutDataTypeStr=uint8
  Cast1 : DataTypeConversion  OutDataTypeStr=uint8
  Cast2 : DataTypeConversion  OutDataTypeStr=uint8
  Constant : Constant  Value=0
  Constant1 : Constant  Value=2
  Constant2 : Constant  Value=2
  Constant3 : Constant  Value=7
  Constant4 : Constant  Value=2
  Display{,1..6} (7 alike) : Display
  Divide : Product  Inputs=*/
  Fix : Rounding  Priority=3  Operator=fix
  Fix1 : Rounding  Priority=6  Operator=fix
  Gain : Gain  Gain=-1
  GreaterThan : RelationalOperator  Priority=2  Operator=<  OutDataTypeStr=boolean  RndMeth=Simplest
  LessThanOrEqual : RelationalOperator  OutDataTypeStr=boolean  RndMeth=Simplest
  LessThanOrEqual1 : RelationalOperator  OutDataTypeStr=boolean  RndMeth=Simplest
  LessThanOrEqual2 : RelationalOperator  Operator=<  OutDataTypeStr=boolean  RndMeth=Simplest
  Minus : Sum  Priority=4  Inputs=-+
  Minus1 : Sum  Priority=4  Inputs=-+
  Multiply : Product
  Plus : Sum  Priority=10  Inputs=+++
  Power : Math  Priority=5  Operator=pow  SaturateOnIntegerOverflow=on
  Power1 : Math  Priority=5  Operator=pow  SaturateOnIntegerOverflow=on
  Power2 : Math  Priority=5  Operator=pow  SaturateOnIntegerOverflow=on
  Switch : Switch  Criteria=u2 > Threshold
  Switch1 : Switch  Criteria=u2 > Threshold
  Switch2 : Switch  Criteria=u2 > Threshold
  coded : Outport
  Overflow : Outport  Port=2
  wires:
  [integer] -> LessThanOrEqual/1, Display5/1
  Switch1/1 -> Switch2/3
  Switch/1 -> Switch2/1
  LessThanOrEqual1/1 -> Switch1/2
  LessThanOrEqual2/1 -> Switch/2, Switch2/2
  magnitude_max/1 -> LessThanOrEqual2/1, Switch/1
  magnitude_min/1 -> Switch1/3, LessThanOrEqual1/2
  magnitude/1 -> Switch/3, LessThanOrEqual2/2, Switch1/1, LessThanOrEqual1/1
  Plus/1 -> Display3/1, coded/1
  LessThanOrEqual/1 -> Overflow/1
  Power2/1 -> LessThanOrEqual/2, Display6/1
  Constant4/1 -> Power2/1
  Minus1/1 -> Power2/2
  Constant3/1 -> Minus1/2
  [prec] -> Power1/2
  Multiply/1 -> Cast1/1
  precision/1 -> Gain/1, Minus1/1, [prec]
  Power1/1 -> Multiply/2
  Constant2/1 -> Power1/1
  Cast2/1 -> Plus/3, Display2/1
  Fix1/1 -> Cast2/1
  Divide/1 -> Fix1/1
  Power/1 -> Divide/2
  Gain/1 -> Power/2
  Constant1/1 -> Power/1
  Cast1/1 -> Plus/2, Display1/1
  Bit Shift/1 -> Plus/1, Display/1
  Cast/1 -> Bit Shift/1
  Minus/1 -> Divide/1
  Fix/1 -> Minus/1, Multiply/1, [integer]
  GreaterThan/1 -> Cast/1
  Abs/1 -> Fix/1, Minus/2
  Switch2/1 -> GreaterThan/1, Abs/1, Display4/1
  Constant/1 -> GreaterThan/2

== system HANcoder_E407_CAN_COMM_TEST/HANcoder STM32 Target - E407-STM32 algorithm/Tx CAN/float2uint4 ==
  precision : Inport
  magnitude : Inport  Port=2
  magnitude_max : Inport  Port=3
  magnitude_min : Inport  Port=4
  Abs : Abs
  Bit Shift : hdlsllib/Logic and Bit Operations/Bit Shift  mode=Shift Left Logical  N=7
      settings: SourceProductName=HDL Coder  SourceProductBaseCode=HD
  Cast : DataTypeConversion  OutDataTypeStr=uint8
  Cast1 : DataTypeConversion  OutDataTypeStr=uint8
  Cast2 : DataTypeConversion  OutDataTypeStr=uint8
  Constant : Constant  Value=0
  Constant1 : Constant  Value=2
  Constant2 : Constant  Value=2
  Constant3 : Constant  Value=7
  Constant4 : Constant  Value=2
  Display{,1..6} (7 alike) : Display
  Divide : Product  Inputs=*/
  Fix : Rounding  Priority=3  Operator=fix
  Fix1 : Rounding  Priority=6  Operator=fix
  Gain : Gain  Gain=-1
  GreaterThan : RelationalOperator  Priority=2  Operator=<  OutDataTypeStr=boolean  RndMeth=Simplest
  LessThanOrEqual : RelationalOperator  OutDataTypeStr=boolean  RndMeth=Simplest
  LessThanOrEqual1 : RelationalOperator  OutDataTypeStr=boolean  RndMeth=Simplest
  LessThanOrEqual2 : RelationalOperator  Operator=<  OutDataTypeStr=boolean  RndMeth=Simplest
  Minus : Sum  Priority=4  Inputs=-+
  Minus1 : Sum  Priority=4  Inputs=-+
  Multiply : Product
  Plus : Sum  Priority=10  Inputs=+++
  Power : Math  Priority=5  Operator=pow  SaturateOnIntegerOverflow=on
  Power1 : Math  Priority=5  Operator=pow  SaturateOnIntegerOverflow=on
  Power2 : Math  Priority=5  Operator=pow  SaturateOnIntegerOverflow=on
  Switch : Switch  Criteria=u2 > Threshold
  Switch1 : Switch  Criteria=u2 > Threshold
  Switch2 : Switch  Criteria=u2 > Threshold
  coded : Outport
  Overflow : Outport  Port=2
  wires:
  Constant/1 -> GreaterThan/2
  Switch2/1 -> Display4/1, Abs/1, GreaterThan/1
  Abs/1 -> Minus/2, Fix/1
  GreaterThan/1 -> Cast/1
  Fix/1 -> [integer], Multiply/1, Minus/1
  Minus/1 -> Divide/1
  Cast/1 -> Bit Shift/1
  Bit Shift/1 -> Display/1, Plus/1
  Cast1/1 -> Display1/1, Plus/2
  Constant1/1 -> Power/1
  Gain/1 -> Power/2
  Power/1 -> Divide/2
  Divide/1 -> Fix1/1
  Fix1/1 -> Cast2/1
  Cast2/1 -> Display2/1, Plus/3
  Constant2/1 -> Power1/1
  Power1/1 -> Multiply/2
  precision/1 -> [prec], Minus1/1, Gain/1
  Multiply/1 -> Cast1/1
  [prec] -> Power1/2
  Constant3/1 -> Minus1/2
  Minus1/1 -> Power2/2
  Constant4/1 -> Power2/1
  Power2/1 -> Display6/1, LessThanOrEqual/2
  LessThanOrEqual/1 -> Overflow/1
  Plus/1 -> coded/1, Display3/1
  magnitude/1 -> LessThanOrEqual1/1, Switch1/1, LessThanOrEqual2/2, Switch/3
  magnitude_min/1 -> LessThanOrEqual1/2, Switch1/3
  magnitude_max/1 -> Switch/1, LessThanOrEqual2/1
  LessThanOrEqual2/1 -> Switch2/2, Switch/2
  LessThanOrEqual1/1 -> Switch1/2
  Switch/1 -> Switch2/1
  Switch1/1 -> Switch2/3
  [integer] -> Display5/1, LessThanOrEqual/1

== system HANcoder_E407_CAN_COMM_TEST/HANcoder STM32 Target - E407-STM32 algorithm/Tx CAN/float2uint5 ==
  precision : Inport
  magnitude : Inport  Port=2
  magnitude_max : Inport  Port=3
  magnitude_min : Inport  Port=4
  Abs : Abs
  Bit Shift : hdlsllib/Logic and Bit Operations/Bit Shift  mode=Shift Left Logical  N=7
      settings: SourceProductName=HDL Coder  SourceProductBaseCode=HD
  Cast : DataTypeConversion  OutDataTypeStr=uint8
  Cast1 : DataTypeConversion  OutDataTypeStr=uint8
  Cast2 : DataTypeConversion  OutDataTypeStr=uint8
  Constant : Constant  Value=0
  Constant1 : Constant  Value=2
  Constant2 : Constant  Value=2
  Constant3 : Constant  Value=7
  Constant4 : Constant  Value=2
  Display{,1..6} (7 alike) : Display
  Divide : Product  Inputs=*/
  Fix : Rounding  Priority=3  Operator=fix
  Fix1 : Rounding  Priority=6  Operator=fix
  Gain : Gain  Gain=-1
  GreaterThan : RelationalOperator  Priority=2  Operator=<  OutDataTypeStr=boolean  RndMeth=Simplest
  LessThanOrEqual : RelationalOperator  OutDataTypeStr=boolean  RndMeth=Simplest
  LessThanOrEqual1 : RelationalOperator  OutDataTypeStr=boolean  RndMeth=Simplest
  LessThanOrEqual2 : RelationalOperator  Operator=<  OutDataTypeStr=boolean  RndMeth=Simplest
  Minus : Sum  Priority=4  Inputs=-+
  Minus1 : Sum  Priority=4  Inputs=-+
  Multiply : Product
  Plus : Sum  Priority=10  Inputs=+++
  Power : Math  Priority=5  Operator=pow  SaturateOnIntegerOverflow=on
  Power1 : Math  Priority=5  Operator=pow  SaturateOnIntegerOverflow=on
  Power2 : Math  Priority=5  Operator=pow  SaturateOnIntegerOverflow=on
  Switch : Switch  Criteria=u2 > Threshold
  Switch1 : Switch  Criteria=u2 > Threshold
  Switch2 : Switch  Criteria=u2 > Threshold
  coded : Outport
  Overflow : Outport  Port=2
  wires:
  [integer] -> LessThanOrEqual/1, Display5/1
  Switch1/1 -> Switch2/3
  Switch/1 -> Switch2/1
  LessThanOrEqual1/1 -> Switch1/2
  LessThanOrEqual2/1 -> Switch/2, Switch2/2
  magnitude_max/1 -> LessThanOrEqual2/1, Switch/1
  magnitude_min/1 -> Switch1/3, LessThanOrEqual1/2
  magnitude/1 -> Switch/3, LessThanOrEqual2/2, Switch1/1, LessThanOrEqual1/1
  Plus/1 -> Display3/1, coded/1
  LessThanOrEqual/1 -> Overflow/1
  Power2/1 -> LessThanOrEqual/2, Display6/1
  Constant4/1 -> Power2/1
  Minus1/1 -> Power2/2
  Constant3/1 -> Minus1/2
  [prec] -> Power1/2
  Multiply/1 -> Cast1/1
  precision/1 -> Gain/1, Minus1/1, [prec]
  Power1/1 -> Multiply/2
  Constant2/1 -> Power1/1
  Cast2/1 -> Plus/3, Display2/1
  Fix1/1 -> Cast2/1
  Divide/1 -> Fix1/1
  Power/1 -> Divide/2
  Gain/1 -> Power/2
  Constant1/1 -> Power/1
  Cast1/1 -> Plus/2, Display1/1
  Bit Shift/1 -> Plus/1, Display/1
  Cast/1 -> Bit Shift/1
  Minus/1 -> Divide/1
  Fix/1 -> Minus/1, Multiply/1, [integer]
  GreaterThan/1 -> Cast/1
  Abs/1 -> Fix/1, Minus/2
  Switch2/1 -> GreaterThan/1, Abs/1, Display4/1
  Constant/1 -> GreaterThan/2
